simulink model "myss_p1_ej1"  (R2022b)
settings: Solver=VariableStepAuto  StartTime=0.0  StopTime=120  RelTol=1e-3
settings Model: Creator=adrub  LastModifiedBy=adrub

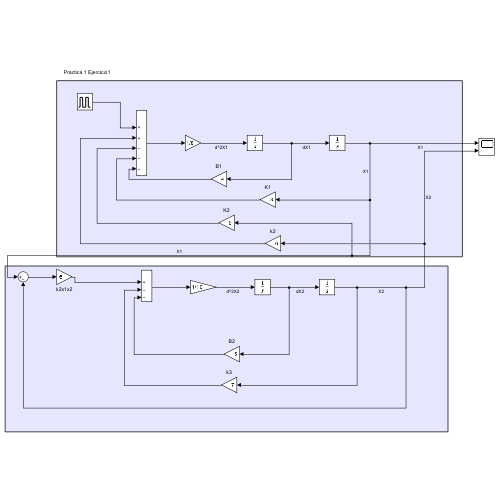
[thumbnail: Simulink's stored preview of the top-level diagram]
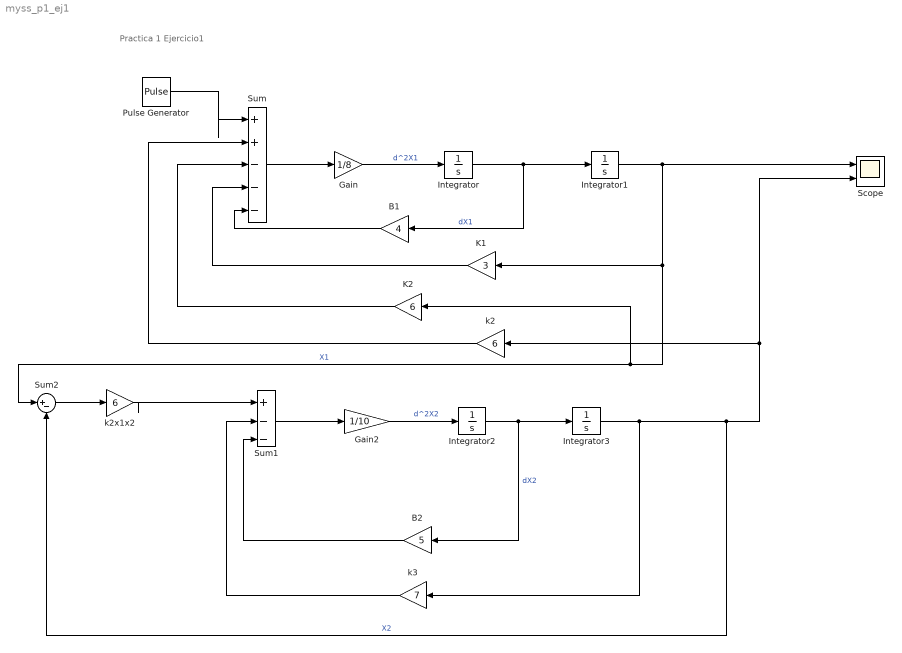
== system myss_p1_ej1 ==
  note: Practica 1 Ejercicio1
  B1 : Gain  Gain=4
  B2 : Gain  Gain=5
  Gain : Gain  Gain=1/8
  Gain2 : Gain  Gain=1/10
  Integrator{,1..3} (4 alike) : Integrator
  K1 : Gain  Gain=3
  K2 : Gain  Gain=6
  Pulse Generator : DiscretePulseGenerator  PulseType=Time based  Period=50  PulseWidth=20
  Scope : Scope  NumInputPorts=2
  Sum : Sum  Inputs=|++---
  Sum1 : Sum  Inputs=|+--
  Sum2 : Sum  Inputs=|+-
  k2 : Gain  Gain=6
  k2x1x2 : Gain  Gain=6
  k3 : Gain  Gain=7
  wires:
  Pulse Generator/1 -> Sum/1
  Sum/1 -> Gain/1
  Gain/1 -> Integrator/1  "d^2X1"
  Integrator/1 -> B1/1, Integrator1/1  "dX1"
  Integrator1/1 -> Sum2/1, K2/1, K1/1, Scope/1  "X1"
  B1/1 -> Sum/5
  K2/1 -> Sum/3
  K1/1 -> Sum/4
  Sum1/1 -> Gain2/1
  Gain2/1 -> Integrator2/1  "d^2X2"
  Integrator2/1 -> B2/1, Integrator3/1  "dX2"
  Integrator3/1 -> k3/1, Sum2/2, k2/1, Scope/2  "X2"
  k2/1 -> Sum/2
  B2/1 -> Sum1/3
  k3/1 -> Sum1/2
  k2x1x2/1 -> Sum1/1
  Sum2/1 -> k2x1x2/1
